simulink model "ISC_laboratorio_02_02"  (R2019a)
settings: Solver=FixedStepAuto  StartTime=0.0  StopTime=200  RelTol=1e-3
undefined symbols (not defined in the file): x0
settings Model: Creator=guilh  LastModifiedBy=guilh
settings DataIOCC: SaveOutput=off  ReturnWorkspaceOutputs=off  StateSaveName=x2  TimeSaveName=t  OutputSaveName=y2

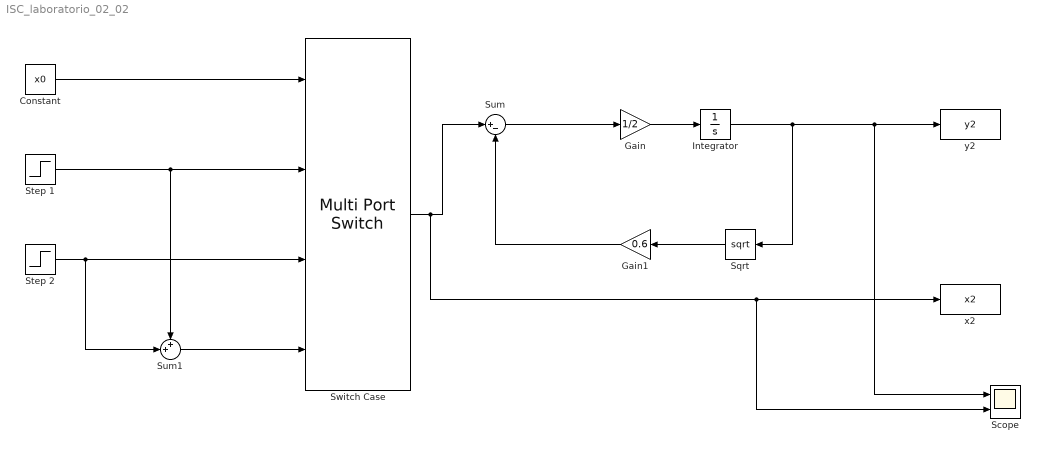
== system ISC_laboratorio_02_02 ==
  Constant : Constant  Value=x0
  Gain : Gain  Gain=1/2
  Gain1 : Gain  Gain=0.6
  Integrator : Integrator
  Scope : Scope  NumInputPorts=2
  Sqrt : Sqrt  SaturateOnIntegerOverflow=on
  Step 1 : Step  Time=0  SampleTime=0
  Step 2 : Step  Time=0  After=2  SampleTime=0
  Sum : Sum  Inputs=|+-
  Sum1 : Sum  Inputs=++|
  Switch Case : MultiPortSwitch
  "x2 " : ToWorkspace  VariableName=x2  SampleTime=-1
  y2 : ToWorkspace  VariableName=y2  SampleTime=-1
  wires:
  Sqrt/1 -> Gain1/1
  Gain1/1 -> Sum/2
  Sum/1 -> Gain/1
  Gain/1 -> Integrator/1
  Integrator/1 -> Scope/1, y2/1, Sqrt/1
  Step 1/1 -> Sum1/1, Switch Case/2
  Constant/1 -> Switch Case/1
  Step 2/1 -> Sum1/2, Switch Case/3
  Sum1/1 -> Switch Case/4
  Switch Case/1 -> Scope/2, "x2 "/1, Sum/1
